simulink model "controlePorVariasSintoniasPI"  (R2023a)
settings: Solver=VariableStepAuto  StartTime=0.0  StopTime=2800  RelTol=1e-3
values from neighbouring files (symbols this model uses):
  F2 = 6.32    [ConstantesCPQ23m.m]    (also in lugardasRaizes.m)
  K = J/(Tau*wn2)    [ConstantesCPQ23m.m]    (also in lugardasRaizes.m)
  qsi = (P/Tau)/(2*wn)    [ConstantesCPQ23m.m]    (also in lugardasRaizes.m)
  wn = sqrt(1/Tau)    [ConstantesCPQ23m.m]    (also in lugardasRaizes.m)
  wn2 = (1/Tau)    [ConstantesCPQ23m.m]    (also in lugardasRaizes.m)
settings Model: Creator=Estudo  LastModifiedBy=Estudo

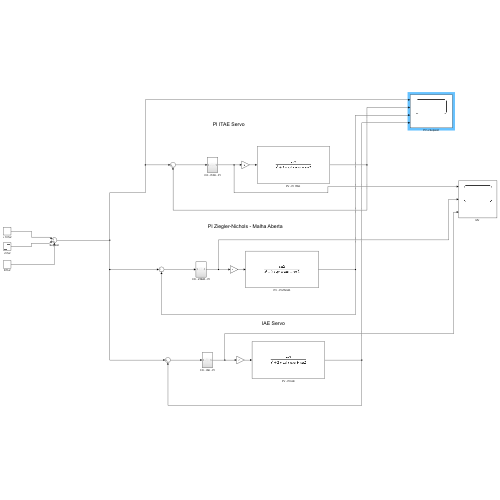
[thumbnail: Simulink's stored preview of the top-level diagram]
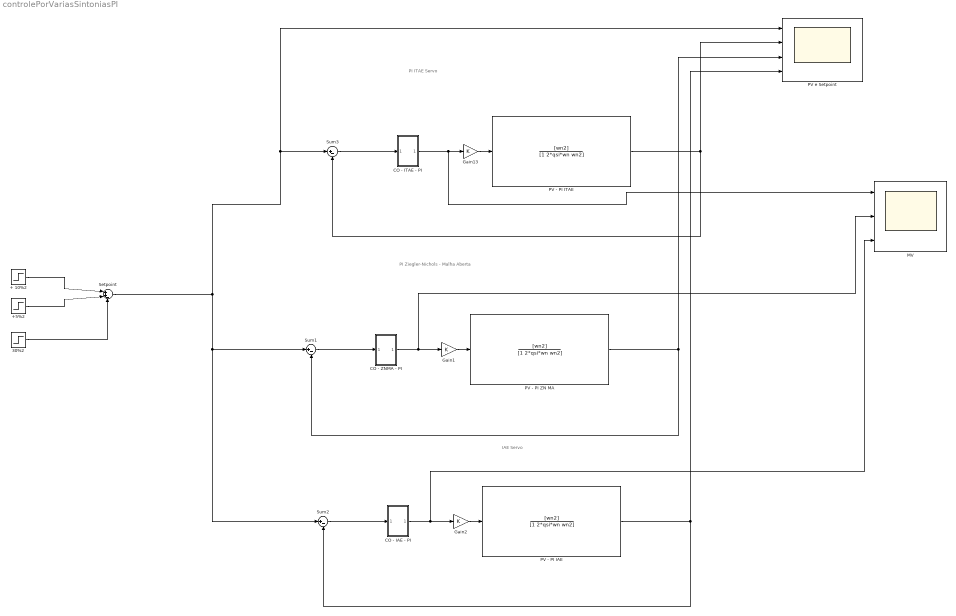
== system controlePorVariasSintoniasPI ==
  note: PI Ziegler-Nichols - Malha Aberta
  note: PI ITAE Servo
  note: IAE Servo
  + 10%2 : Step  After=F2 + F2*0.1  SampleTime=0
  +5%2 : Step  Time=1200  After=F2*0.05  SampleTime=0
  30%2 : Step  Time=2000  After=F2*0.3  SampleTime=0
  CO - IAE - PI : Subsystem
  CO - ITAE - PI : Subsystem
  CO - ZNMA - PI : Subsystem
  Gain1 : Gain  Gain=K
  Gain13 : Gain  Gain=K
  Gain2 : Gain  Gain=K
  "MV " : Scope  NumInputPorts=3
  PV - PI IAE : TransferFcn  Numerator=[wn2]  Denominator=[1 2*qsi*wn wn2]
  "PV - PI ITAE " : TransferFcn  Numerator=[wn2]  Denominator=[1 2*qsi*wn wn2]
  PV - PI ZN MA : TransferFcn  Numerator=[wn2]  Denominator=[1 2*qsi*wn wn2]
  PV e Setpoint : Scope  NumInputPorts=4
  Setpoint : Sum  Inputs=|++-
  Sum1 : Sum  Inputs=|+-
  Sum2 : Sum  Inputs=|+-
  Sum3 : Sum  Inputs=|+-
  wires:
  CO - ITAE - PI/1(Out1) -> "MV "/1, Gain13/1
  Sum3/1 -> CO - ITAE - PI/1(In1)
  Gain13/1 -> "PV - PI ITAE "/1
  "PV - PI ITAE "/1 -> PV e Setpoint/2, Sum3/2
  Setpoint/1 -> PV e Setpoint/1, Sum3/1, Sum2/1, Sum1/1
  Sum1/1 -> CO - ZNMA - PI/1(In1)
  Gain1/1 -> PV - PI ZN MA/1
  PV - PI ZN MA/1 -> PV e Setpoint/3, Sum1/2
  CO - ZNMA - PI/1(Out1) -> "MV "/2, Gain1/1
  + 10%2/1 -> Setpoint/1
  30%2/1 -> Setpoint/3
  +5%2/1 -> Setpoint/2
  PV - PI IAE/1 -> PV e Setpoint/4, Sum2/2
  CO - IAE - PI/1(Out1) -> "MV "/3, Gain2/1
  Sum2/1 -> CO - IAE - PI/1(In1)
  Gain2/1 -> PV - PI IAE/1

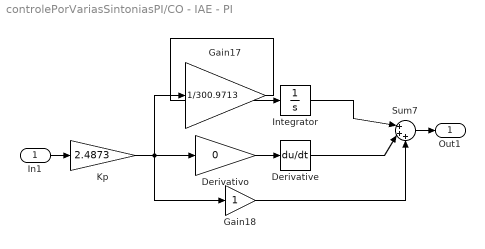
== system controlePorVariasSintoniasPI/CO - IAE - PI ==
  In1 : Inport
  Derivative : Derivative
  Derivativo : Gain  Gain=0
  Gain17 : Gain  Gain=1/300.9713
  Gain18 : Gain
  Integrator : Integrator
  Kp : Gain  Gain=2.4873
  Sum7 : Sum  Inputs=|+++
  Out1 : Outport
  wires:
  Gain18/1 -> Sum7/3
  Integrator/1 -> Sum7/1
  Kp/1 -> Gain17/1, Gain18/1, Derivativo/1
  Derivativo/1 -> Derivative/1
  In1/1 -> Kp/1
  Gain17/1 -> Integrator/1
  Derivative/1 -> Sum7/2
  Sum7/1 -> Out1/1

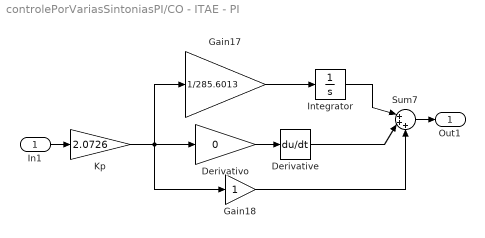
== system controlePorVariasSintoniasPI/CO - ITAE - PI ==
  In1 : Inport
  Derivative : Derivative
  Derivativo : Gain  Gain=0
  Gain17 : Gain  Gain=1/285.6013
  Gain18 : Gain
  Integrator : Integrator
  Kp : Gain  Gain=2.0726
  Sum7 : Sum  Inputs=|+++
  Out1 : Outport
  wires:
  Gain18/1 -> Sum7/3
  Integrator/1 -> Sum7/1
  Kp/1 -> Gain17/1, Gain18/1, Derivativo/1
  Derivativo/1 -> Derivative/1
  In1/1 -> Kp/1
  Gain17/1 -> Integrator/1
  Derivative/1 -> Sum7/2
  Sum7/1 -> Out1/1

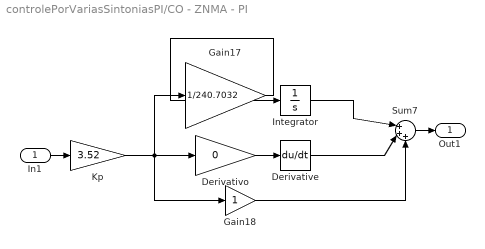
== system controlePorVariasSintoniasPI/CO - ZNMA - PI ==
  In1 : Inport
  Derivative : Derivative
  Derivativo : Gain  Gain=0
  Gain17 : Gain  Gain=1/240.7032
  Gain18 : Gain
  Integrator : Integrator
  Kp : Gain  Gain=3.52
  Sum7 : Sum  Inputs=|+++
  Out1 : Outport
  wires:
  Gain18/1 -> Sum7/3
  Integrator/1 -> Sum7/1
  Kp/1 -> Gain17/1, Gain18/1, Derivativo/1
  Derivativo/1 -> Derivative/1
  In1/1 -> Kp/1
  Gain17/1 -> Integrator/1
  Derivative/1 -> Sum7/2
  Sum7/1 -> Out1/1
